simulink model "HeartRate"  (R2012b)
settings: Solver=FixedStepDiscrete  StartTime=0.0  StopTime=50  RelTol=1e-3
InitFcn:
  | N=256;
  | Fs = 1000;
  | bw = 5.6;
undefined symbols (not defined in the file): gcbh, rmidispblock
settings Model: RequirementInfo={'other' '..\..\..\requirements\ebd_srs.doc' '@Simulink_requirement_heartrate' 'true' '3.1.3.7 Output heartrate from Level 5 QRS complex features This is defined as 1/(Tpeak(n) – Tpeak(n-1)) when peak n is detected, converted to beats per minute. Note that this must be calculated at the original sampling rate to achieve adequate resolution of <=0.1 beats per minute.' '' } %GIDa_a99788a1_c7e6_43a5_a833_a22228035aaa  Creator=aanantha  LastModifiedBy=klindqvi
settings DataIOCC: SaveFormat=Structure  SignalLoggingSaveFormat=ModelDataLogs  SaveOutput=off  SaveTime=off  SignalLoggingName=logsOut
settings OptimizationCC: InlineParams=on  OptimizeModelRefInitCode=on  LifeSpan=1
settings DebuggingCC: ReadBeforeWriteMsg=DisableAll  WriteAfterWriteMsg=DisableAll  WriteAfterReadMsg=DisableAll  SolverPrmCheckMsg=none  InheritedTsInSrcMsg=none  ParameterPrecisionLossMsg=none  FcnCallInpInsideContextMsg=EnableAllAsWarning
settings HardwareCC: ProdLargestAtomicInteger=Long  ProdLargestAtomicFloat=Double  ProdEndianess=LittleEndian  ProdHWDeviceType=ARM Compatible->ARM Cortex
settings RTWCC: SystemTargetFile=ert.tlc  TemplateMakefile=ert_default_tmf  Description=Embedded Coder  GenerateReport=on  RTWVerbose=off  ProcessScript=ert_make_rtw_hook  IncludeHyperlinkInReport=on  LaunchReport=on  PortableWordSizes=on  CodeProfilingSaveOptions=AllData  GenerateTraceInfo=on  GenerateTraceReportSl=on  GenerateTraceReportSf=on  GenerateTraceReportEml=on  GenerateCodeMetricsReport=on
settings CodeAppCC: IgnoreCustomStorageClasses=off
settings ERTTargetCC: CodeReplacementLibrary=GCC ARM Cortex-A8  MultiwordLength=2048  GenerateSampleERTMain=on  ERTCustomFileTemplate=example_file_process.tlc  ConvertIfToSwitch=off  SuppressUnreachableDefaultCases=off

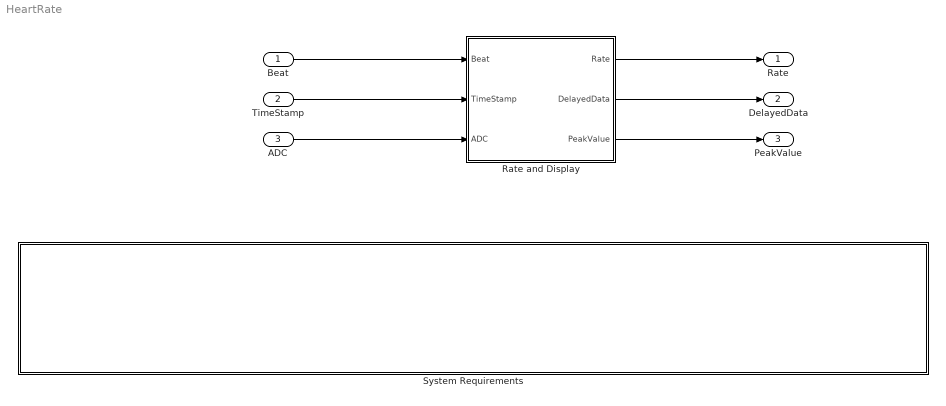
== system HeartRate ==
  Beat : Inport  OutDataTypeStr=boolean  PortDimensions=1  SampleTime=[0.001,0]
  TimeStamp : Inport  Port=2  OutDataTypeStr=uint32  PortDimensions=1  SampleTime=[0.001,0]
  ADC : Inport  Port=3  OutDataTypeStr=single  PortDimensions=1  SampleTime=[0.001,0]
  Rate and Display : Subsystem  RequirementInfo="{'other' '..\\..\\..\\requirements\\ebd_srs.doc' '@3.1.3.8  Output ECG data at input sample rate after processing via a mild low-pass digital filter, delayed to be synchronous with the results of the L5 peak analysis results.' 'true' '3.1.3.8 Output ECG data at input sample rate after processing via a mild low-pass digital filter, delayed to be synchronous with the results of the L5 peak analysis results.' 'Requirement' } %GIDa_44691482_04ec_4835_9d4a_1be8fbf67180"  mask{BuffSize=300}
      mask prompts: BuffSize "Buffer Size"
  System Requirements : Subsystem  LoadFcn=rmidispblock('load',gcbh)  mask(System Requirements){id=SystemReq, title=System Requirements}
      mask prompts: title "Block Title"
      mask help: Lists the requirements for the current model.
      mask init:
      | id = 'SystemReq';
      | [w,h] = rmidispblock('display',gcbh);
      settings: CopyFcn=rmidispblock('create',gcbh)  DeleteFcn=rmidispblock('delete',gcbh)  ModelCloseFcn=rmidispblock('close',gcbh)  PreSaveFcn=rmidispblock('close',gcbh)  PostSaveFcn=rmidispblock('open',gcbh)  OpenFcn=rmidispblock('open',gcbh)  MoveFcn=rmidispblock('move',gcbh)
      mask Help: helpview(fullfile(docroot,'toolbox','slvnv','slvnv.map'),'systemrequirements')
      mask Display: text(w/2,h-4,rmidispblock('title',gcbh),'horizontalAlignment','center','verticalAlignment','top')
  Rate : Outport  OutDataTypeStr=double  PortDimensions=1  SampleTime=[0.001,0]
  DelayedData : Outport  Port=2  OutDataTypeStr=single  PortDimensions=1  SampleTime=[0.001,0]
  PeakValue : Outport  Port=3  OutDataTypeStr=double  PortDimensions=1  SampleTime=[0.001,0]
  wires:
  Rate and Display/1(Rate) -> Rate/1
  TimeStamp/1 -> Rate and Display/2(TimeStamp)
  ADC/1 -> Rate and Display/3(ADC)
  Beat/1 -> Rate and Display/1(Beat)
  Rate and Display/3(PeakValue) -> PeakValue/1
  Rate and Display/2(DelayedData) -> DelayedData/1

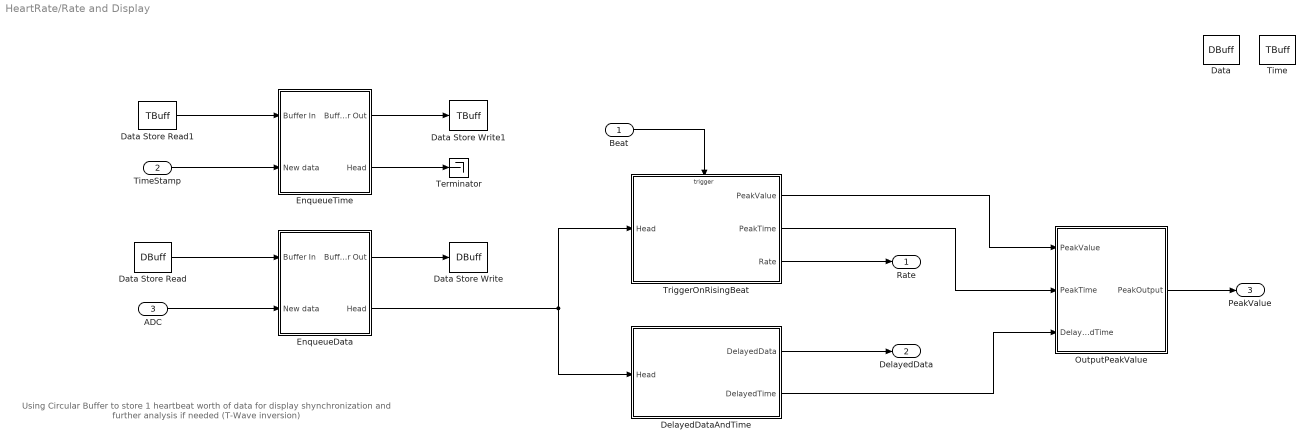
== system HeartRate/Rate and Display ==
  note: Using Circular Buffer to store 1 heartbeat worth of data for
      | display shynchronization and further analysis
      | if needed (T-Wave inversion)
  Beat : Inport
  TimeStamp : Inport  Port=2
  ADC : Inport  Port=3
  Data : DataStoreMemory  DataStoreName=DBuff  ReadBeforeWriteMsg=warning  WriteAfterWriteMsg=warning  WriteAfterReadMsg=warning  InitialValue=zeros(BuffSize,1)
  Data Store Read : DataStoreRead  DataStoreName=DBuff
  Data Store Read1 : DataStoreRead  DataStoreName=TBuff
  Data Store Write : DataStoreWrite  Priority=1  DataStoreName=DBuff
  Data Store Write1 : DataStoreWrite  Priority=2  DataStoreName=TBuff
  DelayedDataAndTime : Subsystem  Priority=5
  EnqueueData : Subsystem
  EnqueueTime : Subsystem
  OutputPeakValue : Subsystem  RequirementInfo={'other' '..\..\..\requirements\ebd_srs.doc' '@Simulink_requirement_peakvalue' 'true' '3.1.3.9 Output a zero for non-R peaks and the peak value for R peaks' '' } %GIDa_f9604a19_3f79_4318_80cf_b6e388b83cfa
  Terminator : Terminator
  Time : DataStoreMemory  DataStoreName=TBuff  ReadBeforeWriteMsg=warning  WriteAfterWriteMsg=warning  WriteAfterReadMsg=warning  InitialValue=zeros(BuffSize,1)
  TriggerOnRisingBeat : Subsystem  Priority=3  TreatAsAtomicUnit=on
  Rate : Outport
  DelayedData : Outport  Port=2
  PeakValue : Outport  Port=3
  wires:
  Beat/1 -> TriggerOnRisingBeat/Trigger
  EnqueueData/1(Buffer Out) -> Data Store Write/1
  ADC/1 -> EnqueueData/2(New data)
  Data Store Read/1 -> EnqueueData/1(Buffer In)
  Data Store Read1/1 -> EnqueueTime/1(Buffer In)
  TimeStamp/1 -> EnqueueTime/2(New data)
  EnqueueTime/1(Buffer Out) -> Data Store Write1/1
  TriggerOnRisingBeat/3(Rate) -> Rate/1
  DelayedDataAndTime/1(DelayedData) -> DelayedData/1
  EnqueueData/2(Head) -> TriggerOnRisingBeat/1(Head), DelayedDataAndTime/1(Head)
  EnqueueTime/2(Head) -> Terminator/1
  TriggerOnRisingBeat/1(PeakValue) -> OutputPeakValue/1(PeakValue)
  TriggerOnRisingBeat/2(PeakTime) -> OutputPeakValue/2(PeakTime)
  DelayedDataAndTime/2(DelayedTime) -> OutputPeakValue/3(DelayedTime)
  OutputPeakValue/1(PeakOutput) -> PeakValue/1

== system HeartRate/System Requirements ==

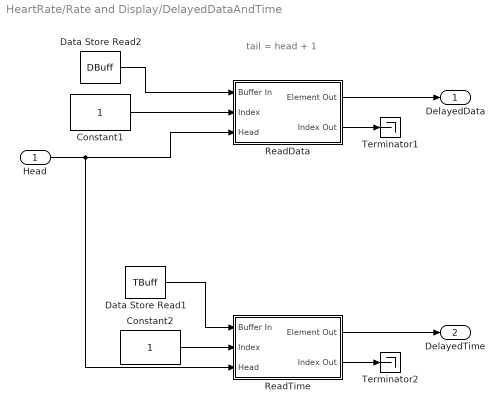
== system HeartRate/Rate and Display/DelayedDataAndTime ==
  note: tail = head + 1
  Head : Inport
  Constant1 : Constant  OutDataTypeStr=int32
  Constant2 : Constant  OutDataTypeStr=int32
  Data Store Read1 : DataStoreRead  DataStoreName=TBuff
  Data Store Read2 : DataStoreRead  DataStoreName=DBuff
  ReadData : Subsystem
  ReadTime : Subsystem
  Terminator1 : Terminator
  Terminator2 : Terminator
  DelayedData : Outport
  DelayedTime : Outport  Port=2
  wires:
  Data Store Read2/1 -> ReadData/1(Buffer In)
  Constant1/1 -> ReadData/2(Index)
  ReadData/1(Element Out) -> DelayedData/1
  Data Store Read1/1 -> ReadTime/1(Buffer In)
  Constant2/1 -> ReadTime/2(Index)
  ReadTime/1(Element Out) -> DelayedTime/1
  Head/1 -> ReadData/3(Head), ReadTime/3(Head)
  ReadData/2(Index Out) -> Terminator1/1
  ReadTime/2(Index Out) -> Terminator2/1

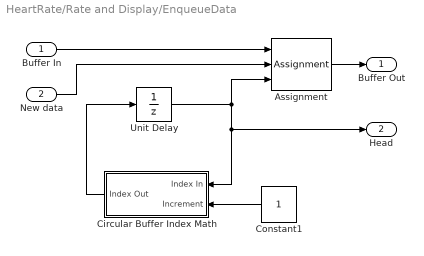
== system HeartRate/Rate and Display/EnqueueData ==
  Buffer In : Inport
  New data : Inport  Port=2
  Assignment : Assignment  IndexOptions=Index vector (port)  Indices=1  OutputSizes=1
  Circular Buffer Index Math : Subsystem
  Constant1 : Constant  OutDataTypeStr=int32
  Unit Delay : UnitDelay  InitialCondition=1  SampleTime=-1
  Buffer Out : Outport
  Head : Outport  Port=2
  wires:
  Constant1/1 -> Circular Buffer Index Math/2(Increment)
  Circular Buffer Index Math/1(Index Out) -> Unit Delay/1
  Unit Delay/1 -> Assignment/3, Circular Buffer Index Math/1(Index In), Head/1
  Buffer In/1 -> Assignment/1
  New data/1 -> Assignment/2
  Assignment/1 -> Buffer Out/1

== system HeartRate/Rate and Display/EnqueueTime ==
  Buffer In : Inport
  New data : Inport  Port=2
  Assignment : Assignment  IndexOptions=Index vector (port)  Indices=1  OutputSizes=1
  Circular Buffer Index Math : Subsystem
  Constant1 : Constant
  Unit Delay : UnitDelay  InitialCondition=1  SampleTime=-1
  Buffer Out : Outport
  Head : Outport  Port=2
  wires:
  Assignment/1 -> Buffer Out/1
  New data/1 -> Assignment/2
  Buffer In/1 -> Assignment/1
  Unit Delay/1 -> Head/1, Circular Buffer Index Math/1(Index In), Assignment/3
  Circular Buffer Index Math/1(Index Out) -> Unit Delay/1
  Constant1/1 -> Circular Buffer Index Math/2(Increment)

== system HeartRate/Rate and Display/OutputPeakValue ==
  PeakValue : Inport
  PeakTime : Inport  Port=2
  DelayedTime : Inport  Port=3
  Constant1 : Constant  Value=0
  Relational Operator : RelationalOperator  Operator===  OutDataTypeStr=boolean
  Switch : Switch  Criteria=u2 ~= 0
  PeakOutput : Outport
  wires:
  PeakTime/1 -> Relational Operator/1
  DelayedTime/1 -> Relational Operator/2
  PeakValue/1 -> Switch/1
  Relational Operator/1 -> Switch/2
  Switch/1 -> PeakOutput/1
  Constant1/1 -> Switch/3

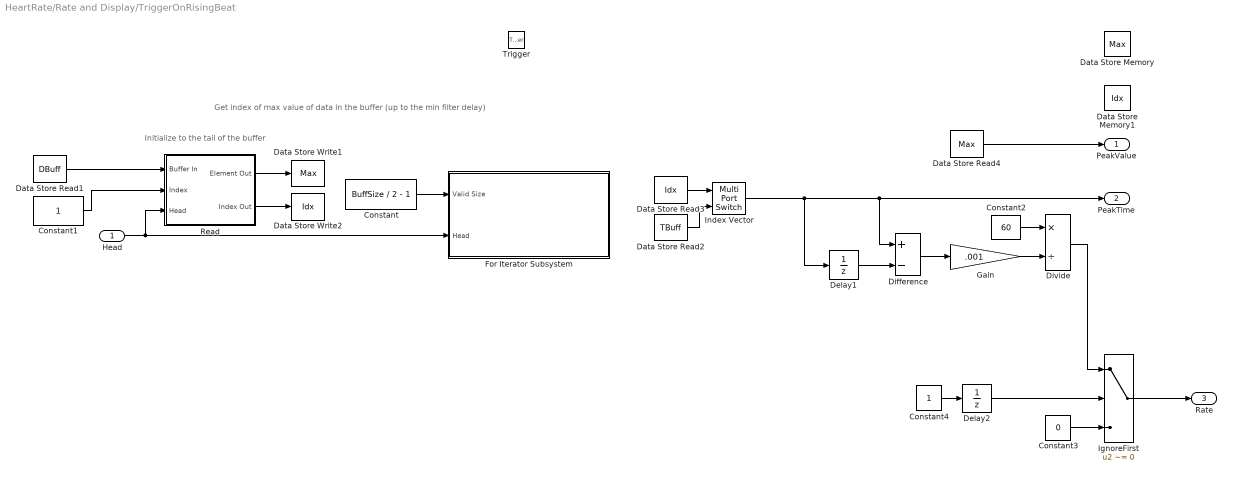
== system HeartRate/Rate and Display/TriggerOnRisingBeat ==
  note: Get index of max value of data in the buffer (up to the min filter delay)
  note: Initialize to the tail of the buffer
  Head : Inport
  Trigger : TriggerPort
  Constant : Constant  Value=BuffSize / 2 - 1  SampleTime=-1
  Constant1 : Constant  SampleTime=-1
  Constant2 : Constant  Value=60  SampleTime=-1
  Constant3 : Constant  Value=0
  Constant4 : Constant
  Data Store Memory : DataStoreMemory  DataStoreName=Max  ReadBeforeWriteMsg=warning  WriteAfterWriteMsg=warning  WriteAfterReadMsg=warning
  Data Store Memory1 : DataStoreMemory  DataStoreName=Idx  ReadBeforeWriteMsg=warning  WriteAfterWriteMsg=warning  WriteAfterReadMsg=warning
  Data Store Read1 : DataStoreRead  DataStoreName=DBuff
  Data Store Read2 : DataStoreRead  Priority=4  DataStoreName=TBuff
  Data Store Read3 : DataStoreRead  Priority=4  DataStoreName=Idx
  Data Store Read4 : DataStoreRead  Priority=4  DataStoreName=Max
  Data Store Write1 : DataStoreWrite  Priority=2  DataStoreName=Max
  Data Store Write2 : DataStoreWrite  Priority=2  DataStoreName=Idx
  Delay1 : UnitDelay  SampleTime=-1
  Delay2 : UnitDelay  SampleTime=-1
  Difference : Sum  Inputs=+-
  Divide : Product  RequirementInfo={'other' '..\..\requirements\ebd_fmea.xlsx' '$B13' 'true' 'B13' 'Risk Management' } %GIDa_07a7caaf_ea0c_45d9_8807_cb91d53ffacc  Inputs=*/
  For Iterator Subsystem : Subsystem  Priority=3  TreatAsAtomicUnit=on
  Gain : Gain  Gain=.001  ParamDataTypeStr=single
  IgnoreFirst : Switch  Criteria=u2 ~= 0
  Index Vector : MultiPortSwitch  Inputs=1
  Read : Subsystem
  PeakValue : Outport
  PeakTime : Outport  Port=2
  Rate : Outport  Port=3
  wires:
  Data Store Read1/1 -> Read/1(Buffer In)
  Read/1(Element Out) -> Data Store Write1/1
  Index Vector/1 -> Delay1/1, PeakTime/1, Difference/1
  Data Store Read4/1 -> PeakValue/1
  Delay1/1 -> Difference/2
  Difference/1 -> Gain/1
  Constant/1 -> For Iterator Subsystem/1(Valid Size)
  Constant1/1 -> Read/2(Index)
  Head/1 -> Read/3(Head), For Iterator Subsystem/2(Head)
  Read/2(Index Out) -> Data Store Write2/1
  Data Store Read3/1 -> Index Vector/1
  Data Store Read2/1 -> Index Vector/2
  Gain/1 -> Divide/2
  Constant2/1 -> Divide/1
  Constant3/1 -> IgnoreFirst/3
  IgnoreFirst/1 -> Rate/1
  Delay2/1 -> IgnoreFirst/2
  Constant4/1 -> Delay2/1
  Divide/1 -> IgnoreFirst/1

== system HeartRate/Rate and Display/DelayedDataAndTime/ReadData ==
  Buffer In : Inport
  Index : Inport  Port=2
  Head : Inport  Port=3
  Circular Buffer Index Math : Subsystem
  Index Vector : MultiPortSwitch  Inputs=1
  Element Out : Outport
  Index Out : Outport  Port=2
  wires:
  Index Vector/1 -> Element Out/1
  Head/1 -> Circular Buffer Index Math/1(Index In)
  Index/1 -> Circular Buffer Index Math/2(Increment)
  Circular Buffer Index Math/1(Index Out) -> Index Vector/1, Index Out/1
  Buffer In/1 -> Index Vector/2

== system HeartRate/Rate and Display/DelayedDataAndTime/ReadTime ==
  Buffer In : Inport
  Index : Inport  Port=2
  Head : Inport  Port=3
  Circular Buffer Index Math : Subsystem
  Index Vector : MultiPortSwitch  Inputs=1
  Element Out : Outport
  Index Out : Outport  Port=2
  wires:
  Buffer In/1 -> Index Vector/2
  Circular Buffer Index Math/1(Index Out) -> Index Out/1, Index Vector/1
  Index/1 -> Circular Buffer Index Math/2(Increment)
  Head/1 -> Circular Buffer Index Math/1(Index In)
  Index Vector/1 -> Element Out/1

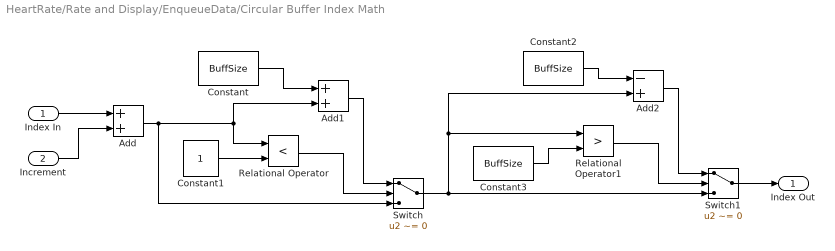
== system HeartRate/Rate and Display/EnqueueData/Circular Buffer Index Math ==
  Index In : Inport
  Increment : Inport  Port=2
  Add : Sum
  Add1 : Sum
  Add2 : Sum  Inputs=-+
  Constant : Constant  Value=BuffSize
  Constant1 : Constant
  Constant2 : Constant  Value=BuffSize
  Constant3 : Constant  Value=BuffSize
  Relational Operator : RelationalOperator  Operator=<  OutDataTypeStr=boolean
  Relational Operator1 : RelationalOperator  Operator=>  OutDataTypeStr=boolean
  Switch : Switch  Criteria=u2 ~= 0
  Switch1 : Switch  Criteria=u2 ~= 0
  Index Out : Outport
  wires:
  Index In/1 -> Add/1
  Increment/1 -> Add/2
  Add/1 -> Relational Operator/1, Add1/2, Switch/3
  Constant1/1 -> Relational Operator/2
  Relational Operator/1 -> Switch/2
  Constant/1 -> Add1/1
  Add1/1 -> Switch/1
  Relational Operator1/1 -> Switch1/2
  Constant2/1 -> Add2/1
  Add2/1 -> Switch1/1
  Constant3/1 -> Relational Operator1/2
  Switch/1 -> Switch1/3, Add2/2, Relational Operator1/1
  Switch1/1 -> Index Out/1

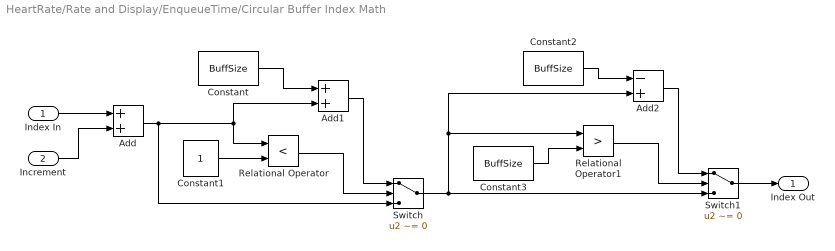
== system HeartRate/Rate and Display/EnqueueTime/Circular Buffer Index Math ==
  Index In : Inport
  Increment : Inport  Port=2
  Add : Sum
  Add1 : Sum
  Add2 : Sum  Inputs=-+
  Constant : Constant  Value=BuffSize
  Constant1 : Constant
  Constant2 : Constant  Value=BuffSize
  Constant3 : Constant  Value=BuffSize
  Relational Operator : RelationalOperator  Operator=<  OutDataTypeStr=boolean
  Relational Operator1 : RelationalOperator  Operator=>  OutDataTypeStr=boolean
  Switch : Switch  Criteria=u2 ~= 0
  Switch1 : Switch  Criteria=u2 ~= 0
  Index Out : Outport
  wires:
  Switch1/1 -> Index Out/1
  Switch/1 -> Relational Operator1/1, Add2/2, Switch1/3
  Constant3/1 -> Relational Operator1/2
  Add2/1 -> Switch1/1
  Constant2/1 -> Add2/1
  Relational Operator1/1 -> Switch1/2
  Add1/1 -> Switch/1
  Constant/1 -> Add1/1
  Relational Operator/1 -> Switch/2
  Constant1/1 -> Relational Operator/2
  Add/1 -> Switch/3, Add1/2, Relational Operator/1
  Increment/1 -> Add/2
  Index In/1 -> Add/1

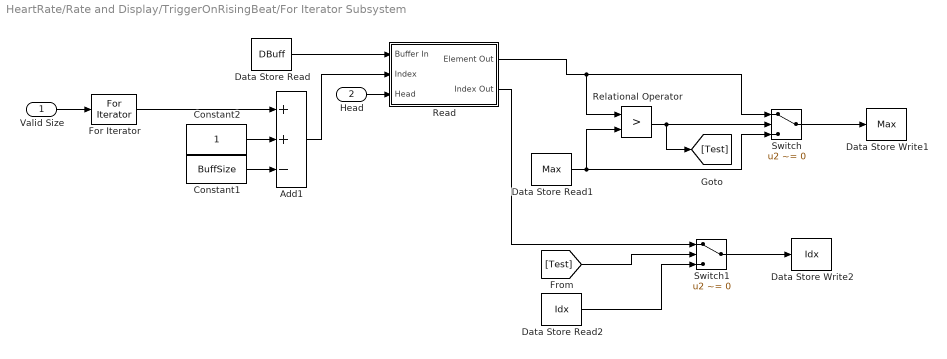
== system HeartRate/Rate and Display/TriggerOnRisingBeat/For Iterator Subsystem ==
  Valid Size : Inport
  Head : Inport  Port=2
  Add1 : Sum  Inputs=++-
  Constant1 : Constant  Value=BuffSize  SampleTime=-1
  Constant2 : Constant  SampleTime=-1
  Data Store Read : DataStoreRead  DataStoreName=DBuff
  Data Store Read1 : DataStoreRead  DataStoreName=Max
  Data Store Read2 : DataStoreRead  DataStoreName=Idx
  Data Store Write1 : DataStoreWrite  Priority=2  DataStoreName=Max
  Data Store Write2 : DataStoreWrite  Priority=2  DataStoreName=Idx
  For Iterator : ForIterator  ResetStates=reset  IterationSource=external
  Read : Subsystem
  Relational Operator : RelationalOperator  Operator=>  OutDataTypeStr=boolean
  Switch : Switch  Criteria=u2 ~= 0
  Switch1 : Switch  Criteria=u2 ~= 0
  wires:
  Data Store Read/1 -> Read/1(Buffer In)
  Read/1(Element Out) -> Switch/1, Relational Operator/1
  For Iterator/1 -> Add1/1
  Data Store Read1/1 -> Switch/3, Relational Operator/2
  Relational Operator/1 -> Switch/2, [Test]
  Switch/1 -> Data Store Write1/1
  Switch1/1 -> Data Store Write2/1
  Data Store Read2/1 -> Switch1/3
  [Test] -> Switch1/2
  Valid Size/1 -> For Iterator/1
  Add1/1 -> Read/2(Index)
  Head/1 -> Read/3(Head)
  Constant2/1 -> Add1/2
  Constant1/1 -> Add1/3
  Read/2(Index Out) -> Switch1/1

== system HeartRate/Rate and Display/TriggerOnRisingBeat/Read ==
  Buffer In : Inport
  Index : Inport  Port=2
  Head : Inport  Port=3
  Circular Buffer Index Math : Subsystem
  Index Vector : MultiPortSwitch  Inputs=1
  Element Out : Outport
  Index Out : Outport  Port=2
  wires:
  Index Vector/1 -> Element Out/1
  Head/1 -> Circular Buffer Index Math/1(Index In)
  Index/1 -> Circular Buffer Index Math/2(Increment)
  Circular Buffer Index Math/1(Index Out) -> Index Vector/1, Index Out/1
  Buffer In/1 -> Index Vector/2

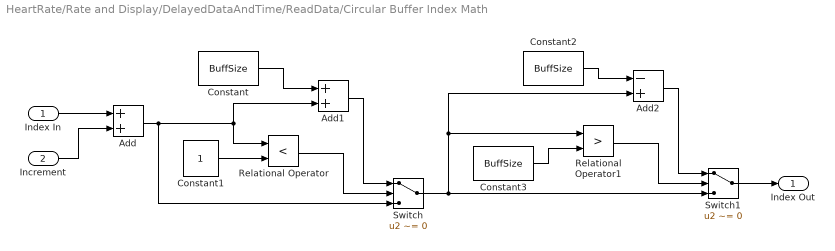
== system HeartRate/Rate and Display/DelayedDataAndTime/ReadData/Circular Buffer Index Math ==
  Index In : Inport
  Increment : Inport  Port=2
  Add : Sum
  Add1 : Sum
  Add2 : Sum  Inputs=-+
  Constant : Constant  Value=BuffSize
  Constant1 : Constant
  Constant2 : Constant  Value=BuffSize
  Constant3 : Constant  Value=BuffSize
  Relational Operator : RelationalOperator  Operator=<  OutDataTypeStr=boolean
  Relational Operator1 : RelationalOperator  Operator=>  OutDataTypeStr=boolean
  Switch : Switch  Criteria=u2 ~= 0
  Switch1 : Switch  Criteria=u2 ~= 0
  Index Out : Outport
  wires:
  Index In/1 -> Add/1
  Increment/1 -> Add/2
  Add/1 -> Relational Operator/1, Add1/2, Switch/3
  Constant1/1 -> Relational Operator/2
  Relational Operator/1 -> Switch/2
  Constant/1 -> Add1/1
  Add1/1 -> Switch/1
  Relational Operator1/1 -> Switch1/2
  Constant2/1 -> Add2/1
  Add2/1 -> Switch1/1
  Constant3/1 -> Relational Operator1/2
  Switch/1 -> Switch1/3, Add2/2, Relational Operator1/1
  Switch1/1 -> Index Out/1

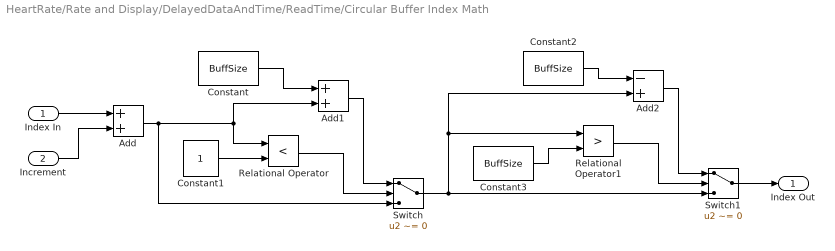
== system HeartRate/Rate and Display/DelayedDataAndTime/ReadTime/Circular Buffer Index Math ==
  Index In : Inport
  Increment : Inport  Port=2
  Add : Sum
  Add1 : Sum
  Add2 : Sum  Inputs=-+
  Constant : Constant  Value=BuffSize
  Constant1 : Constant
  Constant2 : Constant  Value=BuffSize
  Constant3 : Constant  Value=BuffSize
  Relational Operator : RelationalOperator  Operator=<  OutDataTypeStr=boolean
  Relational Operator1 : RelationalOperator  Operator=>  OutDataTypeStr=boolean
  Switch : Switch  Criteria=u2 ~= 0
  Switch1 : Switch  Criteria=u2 ~= 0
  Index Out : Outport
  wires:
  Switch1/1 -> Index Out/1
  Switch/1 -> Relational Operator1/1, Add2/2, Switch1/3
  Constant3/1 -> Relational Operator1/2
  Add2/1 -> Switch1/1
  Constant2/1 -> Add2/1
  Relational Operator1/1 -> Switch1/2
  Add1/1 -> Switch/1
  Constant/1 -> Add1/1
  Relational Operator/1 -> Switch/2
  Constant1/1 -> Relational Operator/2
  Add/1 -> Switch/3, Add1/2, Relational Operator/1
  Increment/1 -> Add/2
  Index In/1 -> Add/1

== system HeartRate/Rate and Display/TriggerOnRisingBeat/For Iterator Subsystem/Read ==
  Buffer In : Inport
  Index : Inport  Port=2
  Head : Inport  Port=3
  Circular Buffer Index Math : Subsystem
  Index Vector : MultiPortSwitch  Inputs=1
  Element Out : Outport
  Index Out : Outport  Port=2
  wires:
  Index Vector/1 -> Element Out/1
  Head/1 -> Circular Buffer Index Math/1(Index In)
  Index/1 -> Circular Buffer Index Math/2(Increment)
  Circular Buffer Index Math/1(Index Out) -> Index Vector/1, Index Out/1
  Buffer In/1 -> Index Vector/2

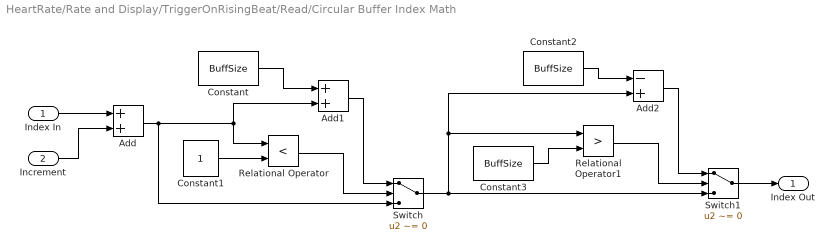
== system HeartRate/Rate and Display/TriggerOnRisingBeat/Read/Circular Buffer Index Math ==
  Index In : Inport
  Increment : Inport  Port=2
  Add : Sum
  Add1 : Sum
  Add2 : Sum  Inputs=-+
  Constant : Constant  Value=BuffSize
  Constant1 : Constant
  Constant2 : Constant  Value=BuffSize
  Constant3 : Constant  Value=BuffSize
  Relational Operator : RelationalOperator  Operator=<  OutDataTypeStr=boolean
  Relational Operator1 : RelationalOperator  Operator=>  OutDataTypeStr=boolean
  Switch : Switch  Criteria=u2 ~= 0
  Switch1 : Switch  Criteria=u2 ~= 0
  Index Out : Outport
  wires:
  Index In/1 -> Add/1
  Increment/1 -> Add/2
  Add/1 -> Relational Operator/1, Add1/2, Switch/3
  Constant1/1 -> Relational Operator/2
  Relational Operator/1 -> Switch/2
  Constant/1 -> Add1/1
  Add1/1 -> Switch/1
  Relational Operator1/1 -> Switch1/2
  Constant2/1 -> Add2/1
  Add2/1 -> Switch1/1
  Constant3/1 -> Relational Operator1/2
  Switch/1 -> Switch1/3, Add2/2, Relational Operator1/1
  Switch1/1 -> Index Out/1

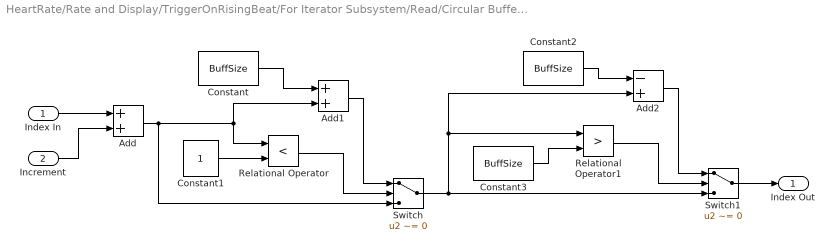
== system HeartRate/Rate and Display/TriggerOnRisingBeat/For Iterator Subsystem/Read/Circular Buffer Index Math ==
  Index In : Inport
  Increment : Inport  Port=2
  Add : Sum
  Add1 : Sum
  Add2 : Sum  Inputs=-+
  Constant : Constant  Value=BuffSize
  Constant1 : Constant
  Constant2 : Constant  Value=BuffSize
  Constant3 : Constant  Value=BuffSize
  Relational Operator : RelationalOperator  Operator=<  OutDataTypeStr=boolean
  Relational Operator1 : RelationalOperator  Operator=>  OutDataTypeStr=boolean
  Switch : Switch  Criteria=u2 ~= 0
  Switch1 : Switch  Criteria=u2 ~= 0
  Index Out : Outport
  wires:
  Index In/1 -> Add/1
  Increment/1 -> Add/2
  Add/1 -> Relational Operator/1, Add1/2, Switch/3
  Constant1/1 -> Relational Operator/2
  Relational Operator/1 -> Switch/2
  Constant/1 -> Add1/1
  Add1/1 -> Switch/1
  Relational Operator1/1 -> Switch1/2
  Constant2/1 -> Add2/1
  Add2/1 -> Switch1/1
  Constant3/1 -> Relational Operator1/2
  Switch/1 -> Switch1/3, Add2/2, Relational Operator1/1
  Switch1/1 -> Index Out/1
